simulink model "OEW_PMSM_180_SVPWM_FOC"  (R2022b)
settings: Solver=FixedStepAuto  StartTime=0.0  StopTime=0.3  FixedStep=Ts  RelTol=1e-3
model workspace (MAT data in the model file):
  B = Simulink.Parameter
  B.Value = 0.002
  B.DataType = 'auto'
  B.Complexity = 'real'
  B.Dimensions = [1 1]
  J = Simulink.Parameter
  J.Value = 0.001
  J.DataType = 'auto'
  J.Complexity = 'real'
  J.Dimensions = [1 1]
  L0 = Simulink.Parameter
  L0.Value = 0.001
  L0.DataType = 'auto'
  L0.Complexity = 'real'
  L0.Dimensions = [1 1]
  Ld = Simulink.Parameter
  Ld.Value = 0.00176
  Ld.DataType = 'auto'
  Ld.Complexity = 'real'
  Ld.Dimensions = [1 1]
  Lq = Simulink.Parameter
  Lq.Value = 0.00176
  Lq.DataType = 'auto'
  Lq.Complexity = 'real'
  Lq.Dimensions = [1 1]
  Rs = Simulink.Parameter
  Rs.Value = 0.2
  Rs.DataType = 'auto'
  Rs.Complexity = 'real'
  Rs.Dimensions = [1 1]
  flux = Simulink.Parameter
  flux.Value = 0.1688
  flux.DataType = 'auto'
  flux.Complexity = 'real'
  flux.Dimensions = [1 1]
  flux_3 = Simulink.Parameter
  flux_3.Value = 0.006
  flux_3.DataType = 'auto'
  flux_3.Complexity = 'real'
  flux_3.Dimensions = [1 1]
  pn = Simulink.Parameter
  pn.Value = 4
  pn.DataType = 'auto'
  pn.Complexity = 'real'
  pn.Dimensions = [1 1]
undefined symbols (not defined in the file): DiscIntNeverNeededParam, Tpwm, Ts, Tsample, Tspeed, Udc
libraries: spsControlledCurrentSourceLib x3, spsVoltageMeasurementLib x3, slpidlib x3, spsUniversalBridgeLib x2, simulink x1, spsDCVoltageSourceLib x1, spsSecondOrderFilterLib x1, sps_lib x1
settings Model: DataDictionary=OEW_PMSM_180_SVPWM_FOC.sldd  Creator=SSC  LastModifiedBy=SSC

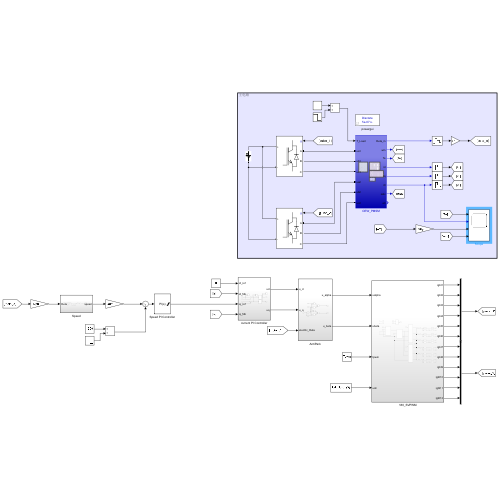
[thumbnail: Simulink's stored preview of the top-level diagram]
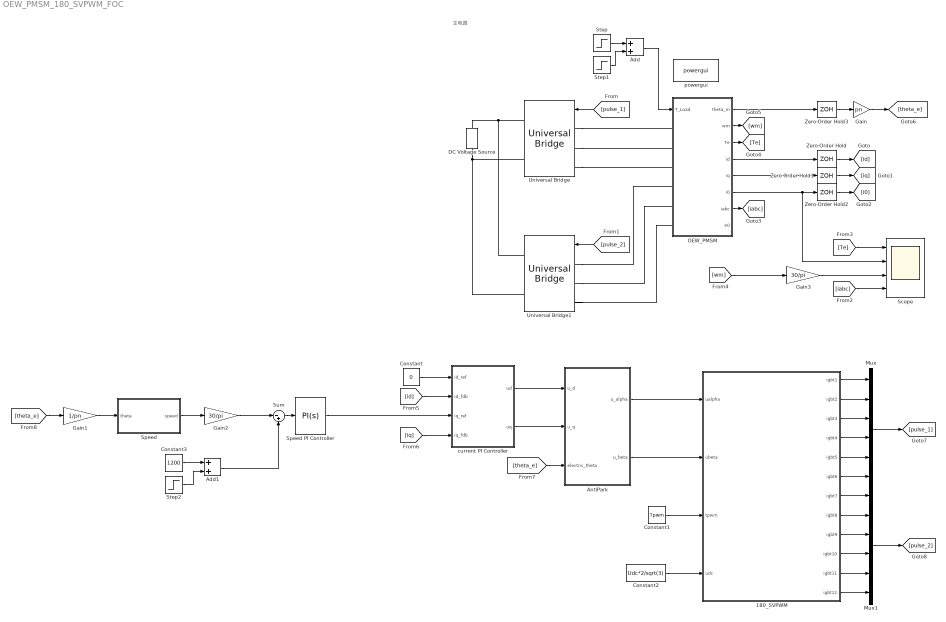
== system OEW_PMSM_180_SVPWM_FOC ==
  note: 主电路
  180_SVPWM : Subsystem
  Add : Sum
  Add1 : Sum
  AntiPark : Subsystem
  Constant : Constant  Value=0
  Constant1 : Constant  Value=Tpwm
  Constant2 : Constant  Value=Udc*2/sqrt(3)
  Constant3 : Constant  Value=1200
  DC Voltage Source : spsDCVoltageSourceLib/DC Voltage Source  Amplitude=Udc  Measurements=None
  Gain : Gain  Gain=pn
  Gain1 : Gain  Gain=1/pn
  Gain2 : Gain  Gain=30/pi
  Gain3 : Gain  Gain=30/pi
  Mux : Mux  Inputs=6
  Mux1 : Mux  Inputs=6
  OEW_PMSM : Subsystem
  Scope : Scope  NumInputPorts=4
  Speed : Subsystem
  Speed PI Controller : slpidlib/PID Controller  Controller=PI  Form=Parallel  TimeDomain=Continuous-time  UseExternalTs=off  SampleTime=1e-4  IntegratorMethod=Forward Euler  FilterMethod=Forward Euler  ControllerParametersSource=internal  P=0.1  I=40  UseKiTs=off  D=0  N=100  UseFilter=on  TunerSelectOption=Transfer Function Based (PID Tuner App)  InitialConditionSource=internal  InitialConditionForIntegrator=0  InitialConditionForFilter=0  DifferentiatorICPrevScaledInput=0  ExternalReset=none  TrackingMode=off  Kt=1  LimitOutput=on  SatLimitsSource=internal  UpperSaturationLimit=14  LowerSaturationLimit=-14  LinearizeAsGain=on  AntiWindupMode=clamping  Kb=1  LimitIntegrator=off  UpperIntegratorSaturationLimit=inf  LowerIntegratorSaturationLimit=-inf  POutMin=[]  POutMax=[]  IOutMin=[]  IOutMax=[]  DOutMin=[]  DOutMax=[]  NOutMin=[]  NOutMax=[]  SumOutMin=[]  SumOutMax=[]  SaturationOutMin=[]  SaturationOutMax=[]  PParamMin=[]  PParamMax=[]  IParamMin=[]  IParamMax=[]  DParamMin=[]  DParamMax=[]  NParamMin=[]  NParamMax=[]  KbParamMin=[]  KbParamMax=[]  KtParamMin=[]  KtParamMax=[]  KbOutMin=[]  KbOutMax=[]  KtOutMin=[]  KtOutMax=[]  IntegratorOutMin=[]  IntegratorOutMax=[]  FilterOutMin=[]  FilterOutMax=[]  SumI1OutMin=[]  SumI1OutMax=[]  SumI2OutMin=[]  SumI2OutMax=[]  SumI3OutMin=[]  SumI3OutMax=[]  SumI4OutMin=[]  SumI4OutMax=[]  SumDOutMin=[]  SumDOutMax=[]  DifferentiatorOutMin=[]  DifferentiatorOutMax=[]  FilterDiffOutCoefMin=[]  FilterDiffOutCoefMax=[]  ReciprocalOutMin=[]  ReciprocalOutMax=[]  SumDenOutMin=[]  SumDenOutMax=[]  SumNumOutMin=[]  SumNumOutMax=[]  DivideOutMin=[]  DivideOutMax=[]  UdiffTsProdOutMin=[]  UdiffTsProdOutMax=[]  NTsProdOutMin=[]  NTsProdOutMax=[]  UintegralTsProdOutMin=[]  UintegralTsProdOutMax=[]  UngainTsProdOutMin=[]  UngainTsProdOutMax=[]  ClampingZeroOutDataTypeStr=Inherit: Inherit via back propagation  ClampingZeroOutMin=[]  ClampingZeroOutMax=[]  FilterDenConstantOutDataTypeStr=Inherit: Inherit via back propagation  FilterDenConstantOutMin=[]  FilterDenConstantOutMax=[]  PCopyOutDataTypeStr=Inherit: Inherit via back propagation  PCopyOutMin=[]  PCopyOutMax=[]  NCopyOutDataTypeStr=Inherit: Inherit via back propagation  NCopyOutMin=[]  NCopyOutMax=[]  IntegratorContinuousStateAttributes=''  IntegratorStateMustResolveToSignalObject=off  IntegratorRTWStateStorageClass=Auto  FilterContinuousStateAttributes=''  FilterStateMustResolveToSignalObject=off  FilterRTWStateStorageClass=Auto  ParallelPVariant=InternalParameters  IdealPVariant=Disabled  IVariant=InternalParameters  DVariant=Disabled  IntegratorVariant=Continuous  SatVariant=Enabled  AWVariant=ContClampingParallel  PCopyVariant=Disabled  TRVariant=Disabled  FdbkBlocksVariant=Forward  IdealPFdbkVariant=Disabled  SatFdbkVariant=Disabled  DerivativeFilterVariant=Disabled  NVariant=Disabled  NCopyVariant=Disabled_SignalSpec  FilterICVariant=Disabled  IntegratorICVariant=InternalICs  ExternalResetVariant=Disabled  TRSumVariant=Passthrough  SumFdbkVariant=Disabled  SumVariant=Sum_PI  TsampFilterVariant=InternalTs  TsampNgainVariant=Passthrough  TsampIntegralVariant=Passthrough  ExternalSaturationOutDataTypeStr=Inherit: Same as second input
  Step : Step  Time=0.05  After=12  SampleTime=0
  Step1 : Step  Time=0.12  After=-6  SampleTime=0
  Step2 : Step  Time=0.15  After=-600  SampleTime=0
  Sum : Sum  Inputs=|-+
  Universal Bridge : spsUniversalBridgeLib/Universal Bridge  Arms=3  SnubberResistance=1e5  SnubberCapacitance=inf  Device=IGBT / Diodes  Ron=1e-3  Lon=0  ForwardVoltages="[  0  0  ]"  ForwardVoltage=0  GTOparameters=[ 10e-6 , 20e-6 ]  IGBTparameters=[ 1e-6 , 2e-6 ]  Measurements=None  Measurements_2=None  converterType=Rectifier
  Universal Bridge1 : spsUniversalBridgeLib/Universal Bridge  Arms=3  SnubberResistance=1e5  SnubberCapacitance=inf  Device=IGBT / Diodes  Ron=1e-3  Lon=0  ForwardVoltages="[  0  0  ]"  ForwardVoltage=0  GTOparameters=[ 10e-6 , 20e-6 ]  IGBTparameters=[ 1e-6 , 2e-6 ]  Measurements=None  Measurements_2=None  converterType=Rectifier
  Zero-Order Hold{,1..3} (4 alike) : ZeroOrderHold  SampleTime=Tsample
  current PI Controller : Subsystem
  powergui : sps_lib/powergui  Priority=1  SimulationMode=Discrete  SampleTime=Ts  frequency=60  Iterations=50  frequencyindice=0  Pbase=100e6  ErrMax=1e-4  UnitsV=kV  UnitsW=MW  buscounter=0  FunctionMessages=off  echomessages=off  EnableUseOfTLC=off  CurrentSourceSwitches=off  DisableSnubberDevices=off  DisableRonSwitches=off  DisableVfSwitches=off  DisplayEquations=off  AutomaticDiscreteSolvers=off  SolverType=Tustin/Backward Euler (TBE)  Interpol=off  ExternalGateDelay=off  methode=off  Ts=100  x0status=blocks  SPID=on  SwTol=0  HookPort=off  NonlinearTolerance=1e-4  nMaxIteration=100  ContinueOnMaxIteration=off  RestoreLinks=warning  ResistiveCurrentMeasurement=off  Frange=[0:2:500]  Ylog=off  Xlog=on  ShowGrid=off  save=off  variable=ZData  structure=0  ZoomFFT=off  StartTime=0.0  cycles=1  DisplayStyle=1  fundamental=60  FreqAxis=off  MaxFrequency=1000  frequencyindicesteady=1  RmsSteady=1  display=off
  wires:
  [pulse_1] -> Universal Bridge/1
  [pulse_2] -> Universal Bridge1/1
  OEW_PMSM/4(id) -> Zero-Order Hold/1
  OEW_PMSM/5(iq) -> Zero-Order Hold1/1
  OEW_PMSM/6(i0) -> Scope/2, Zero-Order Hold2/1
  Zero-Order Hold/1 -> [id]
  Zero-Order Hold1/1 -> [iq]
  Zero-Order Hold2/1 -> [i0]
  OEW_PMSM/7(iabc) -> [iabc]
  [iabc] -> Scope/4
  OEW_PMSM/3(Te) -> [Te]
  [Te] -> Scope/1
  OEW_PMSM/2(wm) -> [wm]
  [wm] -> Gain3/1
  OEW_PMSM/1(theta_m) -> Zero-Order Hold3/1
  Zero-Order Hold3/1 -> Gain/1
  Gain/1 -> [theta_e]
  Step1/1 -> Add/2
  Step/1 -> Add/1
  Add/1 -> OEW_PMSM/1(T_Load)
  Constant/1 -> current PI Controller/1(id_ref)
  [id] -> current PI Controller/2(id_fdb)
  [iq] -> current PI Controller/4(iq_fdb)
  current PI Controller/1(ud) -> AntiPark/1(u_d)
  current PI Controller/2(uq) -> AntiPark/2(u_q)
  [theta_e] -> AntiPark/3(electric_theta)
  AntiPark/1(u_alpha) -> 180_SVPWM/1(ualpha)
  AntiPark/2(u_beta) -> 180_SVPWM/2(ubeta)
  180_SVPWM/5(igbt5) -> Mux/5
  180_SVPWM/6(igbt6) -> Mux/6
  180_SVPWM/4(igbt4) -> Mux/4
  180_SVPWM/3(igbt3) -> Mux/3
  180_SVPWM/2(igbt2) -> Mux/2
  180_SVPWM/1(igbt1) -> Mux/1
  Constant1/1 -> 180_SVPWM/3(tpwm)
  Constant2/1 -> 180_SVPWM/4(udc)
  Mux/1 -> [pulse_1]
  180_SVPWM/7(igbt7) -> Mux1/1
  Mux1/1 -> [pulse_2]
  180_SVPWM/11(igbt11) -> Mux1/5
  180_SVPWM/8(igbt8) -> Mux1/2
  180_SVPWM/10(igbt10) -> Mux1/4
  180_SVPWM/9(igbt9) -> Mux1/3
  180_SVPWM/12(igbt12) -> Mux1/6
  Gain1/1 -> Speed/1(theta)
  [theta_e] -> Gain1/1
  Speed/1(speed) -> Gain2/1
  Gain2/1 -> Sum/1
  Constant3/1 -> Add1/1
  Sum/1 -> Speed PI Controller/1
  Add1/1 -> Sum/2
  Step2/1 -> Add1/2
  Speed PI Controller/1 -> current PI Controller/3(iq_ref)
  Gain3/1 -> Scope/3
  connections:
  Universal Bridge/LConn1 -- OEW_PMSM/LConn1
  Universal Bridge/LConn2 -- OEW_PMSM/LConn2
  Universal Bridge/LConn3 -- OEW_PMSM/LConn3
  Universal Bridge1/LConn1 -- OEW_PMSM/LConn4
  Universal Bridge1/LConn2 -- OEW_PMSM/LConn5
  Universal Bridge1/LConn3 -- OEW_PMSM/LConn6
  DC Voltage Source/LConn1 -- Universal Bridge/RConn2 -- Universal Bridge1/RConn2
  Universal Bridge1/RConn1 -- Universal Bridge/RConn1 -- DC Voltage Source/RConn1

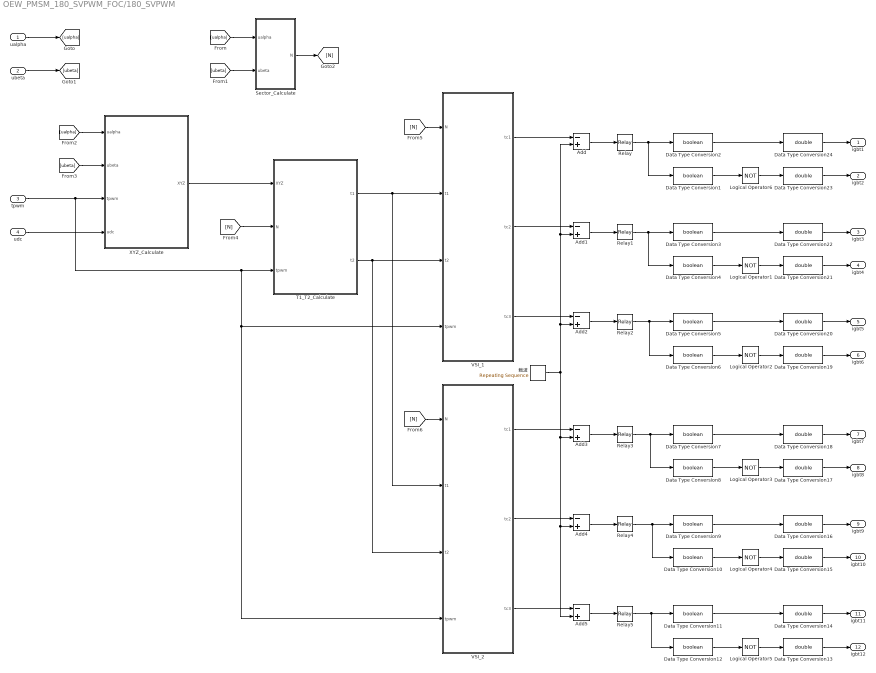
== system OEW_PMSM_180_SVPWM_FOC/180_SVPWM ==
  ualpha : Inport
  ubeta : Inport  Port=2
  tpwm : Inport  Port=3
  udc : Inport  Port=4
  Add{,1..5} (6 alike) : Sum  Inputs=-+
  Data Type Conversion{1..12} (12 alike) : DataTypeConversion  OutDataTypeStr=boolean  SaturateOnIntegerOverflow=off  RndMeth=Floor
  Data Type Conversion{13..24} (12 alike) : DataTypeConversion  OutDataTypeStr=double  SaturateOnIntegerOverflow=off  RndMeth=Floor
  Logical Operator{1..6} (6 alike) : Logic  Operator=NOT  AllPortsSameDT=off  OutDataTypeStr=boolean
  Relay{,1..5} (6 alike) : Relay
  Sector_Calculate : Subsystem
  T1_T2_Calculate : Subsystem
  VSI_1 : Subsystem
  VSI_2 : Subsystem
  XYZ_Calculate : Subsystem
  载波 : simulink/Sources/Repeating Sequence  rep_seq_t=[0 0.5*(1e-4) 1e-4]  rep_seq_y=[0 0.5*(1e-4) 0]
  igbt1 : Outport
  igbt2 : Outport  Port=2
  igbt3 : Outport  Port=3
  igbt4 : Outport  Port=4
  igbt5 : Outport  Port=5
  igbt6 : Outport  Port=6
  igbt7 : Outport  Port=7
  igbt8 : Outport  Port=8
  igbt9 : Outport  Port=9
  igbt10 : Outport  Port=10
  igbt11 : Outport  Port=11
  igbt12 : Outport  Port=12
  wires:
  [ubeta] -> XYZ_Calculate/2(ubeta)
  Relay5/1 -> Data Type Conversion11/1, Data Type Conversion12/1
  Relay2/1 -> Data Type Conversion5/1, Data Type Conversion6/1
  Add2/1 -> Relay2/1
  VSI_1/1(tc1) -> Add/1
  T1_T2_Calculate/2(t2) -> VSI_1/3(t2), VSI_2/3(t2)
  VSI_2/1(tc1) -> Add3/1
  [N] -> VSI_1/1(N)
  Relay1/1 -> Data Type Conversion3/1, Data Type Conversion4/1
  Add3/1 -> Relay3/1
  Add4/1 -> Relay4/1
  Sector_Calculate/1(N) -> [N]
  [ubeta] -> Sector_Calculate/2(ubeta)
  udc/1 -> XYZ_Calculate/4(udc)
  Relay4/1 -> Data Type Conversion9/1, Data Type Conversion10/1
  [N] -> T1_T2_Calculate/2(N)
  载波/1 -> Add/2, Add1/2, Add2/2, Add5/2, Add4/2, Add3/2
  Add/1 -> Relay/1
  [ualpha] -> Sector_Calculate/1(ualpha)
  T1_T2_Calculate/1(t1) -> VSI_1/2(t1), VSI_2/2(t1)
  tpwm/1 -> VSI_2/4(tpwm), VSI_1/4(tpwm), T1_T2_Calculate/3(tpwm), XYZ_Calculate/3(tpwm)
  Logical Operator1/1 -> Data Type Conversion21/1
  Relay/1 -> Data Type Conversion2/1, Data Type Conversion1/1
  XYZ_Calculate/1(XYZ) -> T1_T2_Calculate/1(XYZ)
  Logical Operator2/1 -> Data Type Conversion19/1
  [N] -> VSI_2/1(N)
  Relay3/1 -> Data Type Conversion7/1, Data Type Conversion8/1
  Logical Operator6/1 -> Data Type Conversion23/1
  [ualpha] -> XYZ_Calculate/1(ualpha)
  Logical Operator5/1 -> Data Type Conversion13/1
  Logical Operator4/1 -> Data Type Conversion15/1
  VSI_1/2(tc2) -> Add1/1
  Add5/1 -> Relay5/1
  VSI_2/3(tc3) -> Add5/1
  Add1/1 -> Relay1/1
  VSI_2/2(tc2) -> Add4/1
  VSI_1/3(tc3) -> Add2/1
  Logical Operator3/1 -> Data Type Conversion17/1
  Data Type Conversion2/1 -> Data Type Conversion24/1
  Data Type Conversion1/1 -> Logical Operator6/1
  Data Type Conversion3/1 -> Data Type Conversion22/1
  Data Type Conversion4/1 -> Logical Operator1/1
  Data Type Conversion5/1 -> Data Type Conversion20/1
  Data Type Conversion6/1 -> Logical Operator2/1
  Data Type Conversion7/1 -> Data Type Conversion18/1
  Data Type Conversion8/1 -> Logical Operator3/1
  Data Type Conversion9/1 -> Data Type Conversion16/1
  Data Type Conversion10/1 -> Logical Operator4/1
  Data Type Conversion11/1 -> Data Type Conversion14/1
  Data Type Conversion12/1 -> Logical Operator5/1
  Data Type Conversion13/1 -> igbt12/1
  Data Type Conversion14/1 -> igbt11/1
  Data Type Conversion15/1 -> igbt10/1
  Data Type Conversion16/1 -> igbt9/1
  Data Type Conversion17/1 -> igbt8/1
  Data Type Conversion18/1 -> igbt7/1
  Data Type Conversion19/1 -> igbt6/1
  Data Type Conversion20/1 -> igbt5/1
  Data Type Conversion21/1 -> igbt4/1
  Data Type Conversion22/1 -> igbt3/1
  Data Type Conversion23/1 -> igbt2/1
  Data Type Conversion24/1 -> igbt1/1
  ualpha/1 -> [ualpha]
  ubeta/1 -> [ubeta]

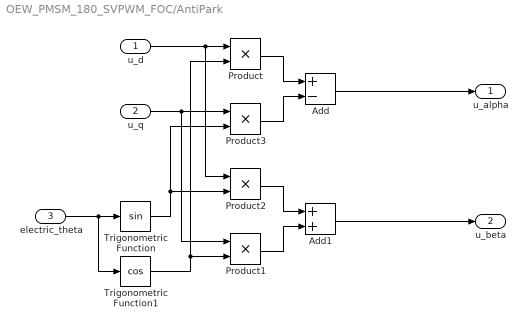
== system OEW_PMSM_180_SVPWM_FOC/AntiPark ==
  u_d : Inport
  u_q : Inport  Port=2
  electric_theta : Inport  Port=3
  Add : Sum  Inputs=+-
  Add1 : Sum
  Product{,1..3} (4 alike) : Product
  Trigonometric Function : Trigonometry
  Trigonometric Function1 : Trigonometry  Operator=cos
  u_alpha : Outport
  u_beta : Outport  Port=2
  wires:
  electric_theta/1 -> Trigonometric Function1/1, Trigonometric Function/1
  u_d/1 -> Product2/1, Product/1
  Trigonometric Function1/1 -> Product/2, Product1/2
  u_q/1 -> Product1/1, Product3/1
  Trigonometric Function/1 -> Product2/2, Product3/2
  Product/1 -> Add/1
  Product3/1 -> Add/2
  Add/1 -> u_alpha/1
  Product2/1 -> Add1/1
  Product1/1 -> Add1/2
  Add1/1 -> u_beta/1

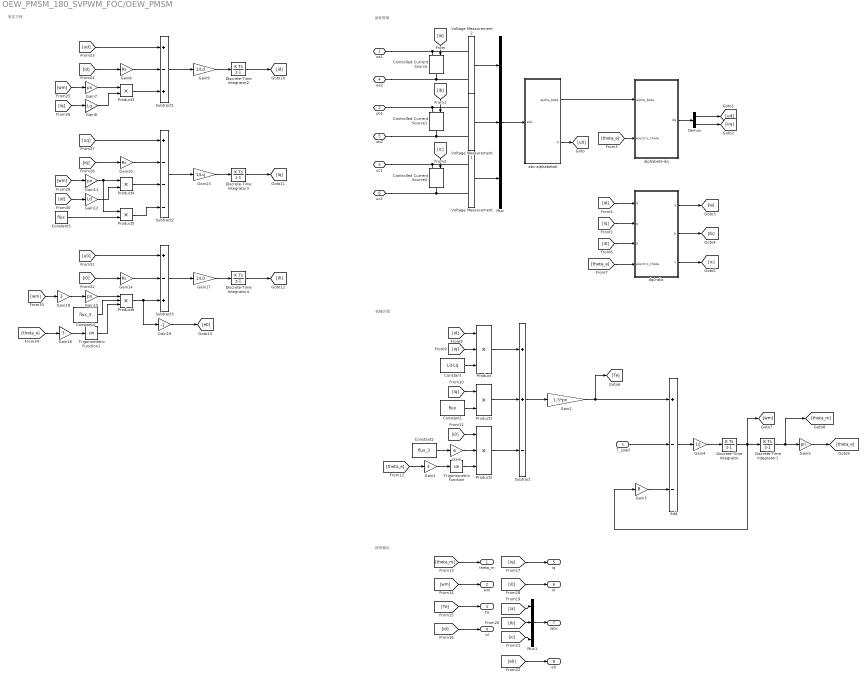
== system OEW_PMSM_180_SVPWM_FOC/OEW_PMSM ==
  note: 电压方程
  note: 信号输出
  note: 机械方程
  note: 坐标变换
  T_Load : Inport
  Add : Sum  Inputs=+--
  Constant : Constant  Value=Ld-Lq
  Constant1 : Constant  Value=flux
  Constant2 : Constant  Value=flux_3
  Constant3 : Constant  Value=flux
  Constant4 : Constant  Value=flux_3
  Controlled Current Source : spsControlledCurrentSourceLib/Controlled Current Source  Initialize=on  Source_Type=AC  Amplitude=0  Phase=0  Frequency=0  Measurements=None
  Controlled Current Source1 : spsControlledCurrentSourceLib/Controlled Current Source  Initialize=on  Source_Type=AC  Amplitude=0  Phase=0  Frequency=0  Measurements=None
  Controlled Current Source2 : spsControlledCurrentSourceLib/Controlled Current Source  Initialize=on  Source_Type=AC  Amplitude=0  Phase=0  Frequency=0  Measurements=None
  Demux : Demux  Outputs=2
  Discrete-Time Integrator{,1..4} (5 alike) : DiscreteIntegrator  SampleTime=Ts  ICPrevOutput=DiscIntNeverNeededParam  ICPrevScaledInput=DiscIntNeverNeededParam
  Gain : Gain  Gain=6
  Gain1 : Gain  Gain=3
  Gain10 : Gain  Gain=Rs
  Gain{5,7,11,15} (4 alike) : Gain  Gain=pn
  Gain12 : Gain  Gain=Ld
  Gain13 : Gain  Gain=1/Lq
  Gain14 : Gain  Gain=Rs
  Gain16 : Gain  Gain=3
  Gain17 : Gain  Gain=1/L0
  Gain18 : Gain  Gain=3
  Gain19 : Gain  Gain=-1
  Gain2 : Gain  Gain=1.5*pn
  Gain3 : Gain  Gain=B
  Gain4 : Gain  Gain=1/J
  Gain6 : Gain  Gain=Rs
  Gain8 : Gain  Gain=Lq
  Gain9 : Gain  Gain=1/Ld
  Mux : Mux  Inputs=3
  Mux1 : Mux  Inputs=3
  Product : Product  Inputs=3
  Product{1,3..5} (4 alike) : Product
  Product2 : Product  Inputs=3
  Product6 : Product  Inputs=3
  Subtract : Sum  Inputs=++-
  Subtract1 : Sum  Inputs=+-+
  Subtract2 : Sum  Inputs=+---
  Subtract3 : Sum  Inputs=+-+
  Trigonometric Function : Trigonometry
  Trigonometric Function1 : Trigonometry
  Voltage Measurement : spsVoltageMeasurementLib/Voltage Measurement  PhasorSimulation=off  OutputType=Complex  PSBequivalent=0
  Voltage Measurement1 : spsVoltageMeasurementLib/Voltage Measurement  PhasorSimulation=off  OutputType=Complex  PSBequivalent=0
  Voltage Measurement2 : spsVoltageMeasurementLib/Voltage Measurement  PhasorSimulation=off  OutputType=Complex  PSBequivalent=0
  abc-alphabeta0 : Subsystem
  alphabeta-dq : Subsystem
  dq0-abc : Subsystem
  ua1 : PMIOPort  Side=Left
  ub1 : PMIOPort  Port=2  Side=Left
  uc1 : PMIOPort  Port=3  Side=Left
  ua2 : PMIOPort  Port=4  Side=Left
  ub2 : PMIOPort  Port=5  Side=Left
  uc2 : PMIOPort  Port=6  Side=Left
  theta_m : Outport
  wm : Outport  Port=2
  Te : Outport  Port=3
  id : Outport  Port=4
  iq : Outport  Port=5
  i0 : Outport  Port=6
  iabc : Outport  Port=7
  e0 : Outport  Port=8
  wires:
  [id] -> Gain12/1
  [id] -> Product/1
  [iq] -> Product/2
  [i0] -> Gain14/1
  alphabeta-dq/1(dq) -> Demux/1
  Gain12/1 -> Product4/2
  Gain19/1 -> [e0]
  [ia] -> Mux1/1
  [iq] -> Gain8/1
  abc-alphabeta0/1(alpha_beta) -> alphabeta-dq/1(alpha_beta)
  Product3/1 -> Subtract1/3
  Subtract2/1 -> Gain13/1
  Gain6/1 -> Subtract1/2
  Product1/1 -> Subtract/2
  Demux/1 -> [ud]
  [theta_e] -> alphabeta-dq/2(electric_theta)
  Gain13/1 -> Discrete-Time Integrator3/1
  Constant1/1 -> Product1/2
  Subtract1/1 -> Gain9/1
  Voltage Measurement1/1 -> Mux/2
  Gain11/1 -> Product5/1, Product4/1
  [ic] -> Controlled Current Source2/1
  dq0-abc/1(a) -> [ia]
  Mux/1 -> abc-alphabeta0/1(abc)
  [iq] -> Gain10/1
  Gain4/1 -> Discrete-Time Integrator/1
  [ib] -> Controlled Current Source1/1
  Demux/2 -> [uq]
  [theta_e] -> Gain16/1
  [ic] -> Mux1/3
  Voltage Measurement/1 -> Mux/3
  Gain3/1 -> Add/3
  Product4/1 -> Subtract2/3
  [iq] -> iq/1
  Gain16/1 -> Trigonometric Function1/1
  [ia] -> Controlled Current Source/1
  Gain1/1 -> Trigonometric Function/1
  abc-alphabeta0/2(0) -> [u0]
  dq0-abc/3(c) -> [ic]
  dq0-abc/2(b) -> [ib]
  T_Load/1 -> Add/2
  [ud] -> Subtract1/1
  Discrete-Time Integrator3/1 -> [iq]
  Voltage Measurement2/1 -> Mux/1
  Constant3/1 -> Product5/2
  Subtract3/1 -> Gain17/1
  Constant/1 -> Product/3
  [iq] -> dq0-abc/2(q)
  [uq] -> Subtract2/1
  Add/1 -> Gain4/1
  [theta_e] -> dq0-abc/4(electric_theta)
  [i0] -> dq0-abc/3(0)
  Product6/1 -> Subtract3/3, Gain19/1
  [id] -> dq0-abc/1(d)
  [wm] -> wm/1
  Discrete-Time Integrator/1 -> Discrete-Time Integrator1/1, Gain3/1, [wm]
  [iq] -> Product1/1
  [wm] -> Gain7/1
  Product/1 -> Subtract/1
  Gain10/1 -> Subtract2/2
  [wm] -> Gain11/1
  Product5/1 -> Subtract2/4
  Constant4/1 -> Product6/2
  Mux1/1 -> iabc/1
  Gain18/1 -> Gain15/1
  Gain5/1 -> [theta_e]
  Trigonometric Function1/1 -> Product6/3
  Gain9/1 -> Discrete-Time Integrator2/1
  Gain7/1 -> Product3/1
  Trigonometric Function/1 -> Product2/3
  Discrete-Time Integrator1/1 -> Gain5/1, [theta_m]
  [ib] -> Mux1/2
  [theta_e] -> Gain1/1
  Gain8/1 -> Product3/2
  [Te] -> Te/1
  Product2/1 -> Subtract/3
  [i0] -> Product2/1
  Discrete-Time Integrator2/1 -> [id]
  [id] -> Gain6/1
  Gain/1 -> Product2/2
  Gain2/1 -> Add/1, [Te]
  Constant2/1 -> Gain/1
  Subtract/1 -> Gain2/1
  [theta_m] -> theta_m/1
  Discrete-Time Integrator4/1 -> [i0]
  Gain17/1 -> Discrete-Time Integrator4/1
  Gain15/1 -> Product6/1
  [u0] -> Subtract3/1
  Gain14/1 -> Subtract3/2
  [wm] -> Gain18/1
  [i0] -> i0/1
  [id] -> id/1
  [e0] -> e0/1
  connections:
  Voltage Measurement2/LConn2 -- ua2/RConn1 -- Controlled Current Source/RConn1
  Voltage Measurement1/LConn2 -- ub2/RConn1 -- Controlled Current Source1/RConn1
  Voltage Measurement2/LConn1 -- ua1/RConn1 -- Controlled Current Source/LConn1
  Voltage Measurement/LConn2 -- uc2/RConn1 -- Controlled Current Source2/RConn1
  Voltage Measurement1/LConn1 -- ub1/RConn1 -- Controlled Current Source1/LConn1
  Voltage Measurement/LConn1 -- uc1/RConn1 -- Controlled Current Source2/LConn1

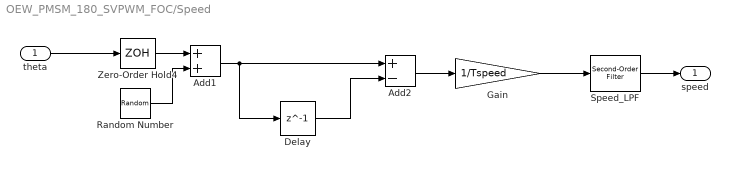
== system OEW_PMSM_180_SVPWM_FOC/Speed ==
  theta : Inport
  Add1 : Sum
  Add2 : Sum  Inputs=+-
  Delay : Delay  DelayLength=1  InitialCondition=0  SampleTime=Tspeed
  Gain : Gain  Gain=1/Tspeed
  Random Number : RandomNumber  Mean=2.5e-10  Variance=2.5e-10  SampleTime=Tspeed
  Speed_LPF : spsSecondOrderFilterLib/Second-Order Filter  FilterType=Lowpass  Fo=500  Zeta=0.707  Ts=Tspeed  Initialize=off  Vac_Init="[0,  0,  60]"  Vdc_Init=0  PlotResponse=off  FreqRange=[0, 500, 1]
      settings: LibrarySourceBlock=|
      | sps_lib/Control/Filters/Second-Order
      | Filter
  Zero-Order Hold4 : ZeroOrderHold  SampleTime=Tspeed
  speed : Outport
  wires:
  Zero-Order Hold4/1 -> Add1/1
  Random Number/1 -> Add1/2
  theta/1 -> Zero-Order Hold4/1
  Speed_LPF/1 -> speed/1
  Add2/1 -> Gain/1
  Gain/1 -> Speed_LPF/1
  Add1/1 -> Delay/1, Add2/1
  Delay/1 -> Add2/2

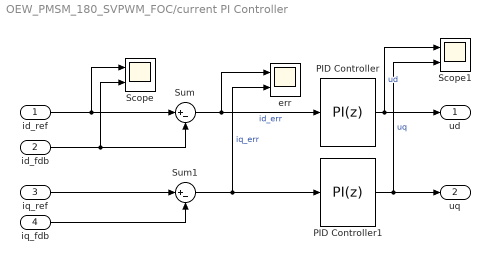
== system OEW_PMSM_180_SVPWM_FOC/current PI Controller ==
  id_ref : Inport
  id_fdb : Inport  Port=2
  iq_ref : Inport  Port=3
  iq_fdb : Inport  Port=4
  PID Controller : slpidlib/PID Controller  Controller=PI  Form=Parallel  TimeDomain=Discrete-time  UseExternalTs=off  SampleTime=Tsample  IntegratorMethod=Forward Euler  FilterMethod=Forward Euler  ControllerParametersSource=internal  P=5.5292  I=628.32  UseKiTs=off  D=0  N=100  UseFilter=on  TunerSelectOption=Transfer Function Based (PID Tuner App)  InitialConditionSource=internal  InitialConditionForIntegrator=0  InitialConditionForFilter=0  DifferentiatorICPrevScaledInput=0  ExternalReset=none  TrackingMode=off  Kt=1  LimitOutput=on  SatLimitsSource=internal  UpperSaturationLimit=Udc  LowerSaturationLimit=-Udc  LinearizeAsGain=on  AntiWindupMode=clamping  Kb=1  LimitIntegrator=off  UpperIntegratorSaturationLimit=inf  LowerIntegratorSaturationLimit=-inf  POutMin=[]  POutMax=[]  IOutMin=[]  IOutMax=[]  DOutMin=[]  DOutMax=[]  NOutMin=[]  NOutMax=[]  SumOutMin=[]  SumOutMax=[]  SaturationOutMin=[]  SaturationOutMax=[]  PParamMin=[]  PParamMax=[]  IParamMin=[]  IParamMax=[]  DParamMin=[]  DParamMax=[]  NParamMin=[]  NParamMax=[]  KbParamMin=[]  KbParamMax=[]  KtParamMin=[]  KtParamMax=[]  KbOutMin=[]  KbOutMax=[]  KtOutMin=[]  KtOutMax=[]  IntegratorOutMin=[]  IntegratorOutMax=[]  FilterOutMin=[]  FilterOutMax=[]  SumI1OutMin=[]  SumI1OutMax=[]  SumI2OutMin=[]  SumI2OutMax=[]  SumI3OutMin=[]  SumI3OutMax=[]  SumI4OutMin=[]  SumI4OutMax=[]  SumDOutMin=[]  SumDOutMax=[]  DifferentiatorOutMin=[]  DifferentiatorOutMax=[]  FilterDiffOutCoefMin=[]  FilterDiffOutCoefMax=[]  ReciprocalOutMin=[]  ReciprocalOutMax=[]  SumDenOutMin=[]  SumDenOutMax=[]  SumNumOutMin=[]  SumNumOutMax=[]  DivideOutMin=[]  DivideOutMax=[]  UdiffTsProdOutMin=[]  UdiffTsProdOutMax=[]  NTsProdOutMin=[]  NTsProdOutMax=[]  UintegralTsProdOutMin=[]  UintegralTsProdOutMax=[]  UngainTsProdOutMin=[]  UngainTsProdOutMax=[]  ClampingZeroOutDataTypeStr=Inherit: Inherit via back propagation  ClampingZeroOutMin=[]  ClampingZeroOutMax=[]  FilterDenConstantOutDataTypeStr=Inherit: Inherit via back propagation  FilterDenConstantOutMin=[]  FilterDenConstantOutMax=[]  PCopyOutDataTypeStr=Inherit: Inherit via back propagation  PCopyOutMin=[]  PCopyOutMax=[]  NCopyOutDataTypeStr=Inherit: Inherit via back propagation  NCopyOutMin=[]  NCopyOutMax=[]  IntegratorContinuousStateAttributes=''  IntegratorStateMustResolveToSignalObject=off  IntegratorRTWStateStorageClass=Auto  FilterContinuousStateAttributes=''  FilterStateMustResolveToSignalObject=off  FilterRTWStateStorageClass=Auto  ParallelPVariant=InternalParameters  IdealPVariant=Disabled  IVariant=InternalParameters  DVariant=Disabled  IntegratorVariant=Discrete  SatVariant=Enabled  AWVariant=DiscClampingParallel  PCopyVariant=Disabled  TRVariant=Disabled  FdbkBlocksVariant=Forward  IdealPFdbkVariant=Disabled  SatFdbkVariant=Disabled  DerivativeFilterVariant=Disabled  NVariant=Disabled  NCopyVariant=Disabled_SignalSpec  FilterICVariant=Disabled  IntegratorICVariant=InternalICs  ExternalResetVariant=Disabled  TRSumVariant=Passthrough  SumFdbkVariant=Disabled  SumVariant=Sum_PI  TsampFilterVariant=InternalTs  TsampNgainVariant=Passthrough  TsampIntegralVariant=Passthrough  ExternalSaturationOutDataTypeStr=Inherit: Same as second input
  PID Controller1 : slpidlib/PID Controller  Controller=PI  Form=Parallel  TimeDomain=Discrete-time  UseExternalTs=off  SampleTime=Tsample  IntegratorMethod=Forward Euler  FilterMethod=Forward Euler  ControllerParametersSource=internal  P=5.5292  I=628.32  UseKiTs=off  D=0  N=100  UseFilter=on  TunerSelectOption=Transfer Function Based (PID Tuner App)  InitialConditionSource=internal  InitialConditionForIntegrator=0  InitialConditionForFilter=0  DifferentiatorICPrevScaledInput=0  ExternalReset=none  TrackingMode=off  Kt=1  LimitOutput=on  SatLimitsSource=internal  UpperSaturationLimit=Udc  LowerSaturationLimit=-Udc  LinearizeAsGain=on  AntiWindupMode=clamping  Kb=1  LimitIntegrator=off  UpperIntegratorSaturationLimit=inf  LowerIntegratorSaturationLimit=-inf  POutMin=[]  POutMax=[]  IOutMin=[]  IOutMax=[]  DOutMin=[]  DOutMax=[]  NOutMin=[]  NOutMax=[]  SumOutMin=[]  SumOutMax=[]  SaturationOutMin=[]  SaturationOutMax=[]  PParamMin=[]  PParamMax=[]  IParamMin=[]  IParamMax=[]  DParamMin=[]  DParamMax=[]  NParamMin=[]  NParamMax=[]  KbParamMin=[]  KbParamMax=[]  KtParamMin=[]  KtParamMax=[]  KbOutMin=[]  KbOutMax=[]  KtOutMin=[]  KtOutMax=[]  IntegratorOutMin=[]  IntegratorOutMax=[]  FilterOutMin=[]  FilterOutMax=[]  SumI1OutMin=[]  SumI1OutMax=[]  SumI2OutMin=[]  SumI2OutMax=[]  SumI3OutMin=[]  SumI3OutMax=[]  SumI4OutMin=[]  SumI4OutMax=[]  SumDOutMin=[]  SumDOutMax=[]  DifferentiatorOutMin=[]  DifferentiatorOutMax=[]  FilterDiffOutCoefMin=[]  FilterDiffOutCoefMax=[]  ReciprocalOutMin=[]  ReciprocalOutMax=[]  SumDenOutMin=[]  SumDenOutMax=[]  SumNumOutMin=[]  SumNumOutMax=[]  DivideOutMin=[]  DivideOutMax=[]  UdiffTsProdOutMin=[]  UdiffTsProdOutMax=[]  NTsProdOutMin=[]  NTsProdOutMax=[]  UintegralTsProdOutMin=[]  UintegralTsProdOutMax=[]  UngainTsProdOutMin=[]  UngainTsProdOutMax=[]  ClampingZeroOutDataTypeStr=Inherit: Inherit via back propagation  ClampingZeroOutMin=[]  ClampingZeroOutMax=[]  FilterDenConstantOutDataTypeStr=Inherit: Inherit via back propagation  FilterDenConstantOutMin=[]  FilterDenConstantOutMax=[]  PCopyOutDataTypeStr=Inherit: Inherit via back propagation  PCopyOutMin=[]  PCopyOutMax=[]  NCopyOutDataTypeStr=Inherit: Inherit via back propagation  NCopyOutMin=[]  NCopyOutMax=[]  IntegratorContinuousStateAttributes=''  IntegratorStateMustResolveToSignalObject=off  IntegratorRTWStateStorageClass=Auto  FilterContinuousStateAttributes=''  FilterStateMustResolveToSignalObject=off  FilterRTWStateStorageClass=Auto  ParallelPVariant=InternalParameters  IdealPVariant=Disabled  IVariant=InternalParameters  DVariant=Disabled  IntegratorVariant=Discrete  SatVariant=Enabled  AWVariant=DiscClampingParallel  PCopyVariant=Disabled  TRVariant=Disabled  FdbkBlocksVariant=Forward  IdealPFdbkVariant=Disabled  SatFdbkVariant=Disabled  DerivativeFilterVariant=Disabled  NVariant=Disabled  NCopyVariant=Disabled_SignalSpec  FilterICVariant=Disabled  IntegratorICVariant=InternalICs  ExternalResetVariant=Disabled  TRSumVariant=Passthrough  SumFdbkVariant=Disabled  SumVariant=Sum_PI  TsampFilterVariant=InternalTs  TsampNgainVariant=Passthrough  TsampIntegralVariant=Passthrough  ExternalSaturationOutDataTypeStr=Inherit: Same as second input
  Scope : Scope  NumInputPorts=2
  Scope1 : Scope  NumInputPorts=2
  Sum : Sum  Inputs=|+-
  Sum1 : Sum  Inputs=|+-
  err : Scope  NumInputPorts=2
  ud : Outport
  uq : Outport  Port=2
  wires:
  iq_fdb/1 -> Sum1/2
  Sum1/1 -> PID Controller1/1, err/2  "iq_err"
  id_fdb/1 -> Scope/2, Sum/2
  Sum/1 -> err/1, PID Controller/1  "id_err"
  id_ref/1 -> Scope/1, Sum/1
  iq_ref/1 -> Sum1/1
  PID Controller1/1 -> Scope1/2, uq/1  "uq"
  PID Controller/1 -> Scope1/1, ud/1  "ud"

== system OEW_PMSM_180_SVPWM_FOC/180_SVPWM/Sector_Calculate ==
  ualpha : Inport
  ubeta : Inport  Port=2
  MATLAB Function : MATLAB Function  TreatAsAtomicUnit=on
  N : Outport
  wires:
  ualpha/1 -> MATLAB Function/1(ualpha)
  ubeta/1 -> MATLAB Function/2(ubeta)
  MATLAB Function/1(N) -> N/1

== system OEW_PMSM_180_SVPWM_FOC/180_SVPWM/T1_T2_Calculate ==
  XYZ : Inport
  N : Inport  Port=2
  tpwm : Inport  Port=3
  Demux : Demux  Outputs=3
  MATLAB Function : MATLAB Function  TreatAsAtomicUnit=on
  t1 : Outport
  t2 : Outport  Port=2
  wires:
  Demux/2 -> MATLAB Function/2(Y)
  Demux/1 -> MATLAB Function/1(X)
  Demux/3 -> MATLAB Function/3(Z)
  XYZ/1 -> Demux/1
  N/1 -> MATLAB Function/4(N)
  tpwm/1 -> MATLAB Function/5(tpwm)
  MATLAB Function/1(t1) -> t1/1
  MATLAB Function/2(t2) -> t2/1

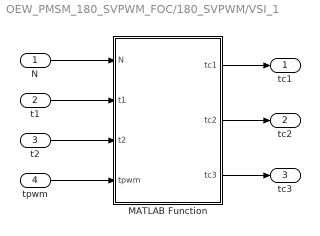
== system OEW_PMSM_180_SVPWM_FOC/180_SVPWM/VSI_1 ==
  N : Inport
  t1 : Inport  Port=2
  t2 : Inport  Port=3
  tpwm : Inport  Port=4
  MATLAB Function : MATLAB Function  TreatAsAtomicUnit=on
  tc1 : Outport
  tc2 : Outport  Port=2
  tc3 : Outport  Port=3
  wires:
  t2/1 -> MATLAB Function/3(t2)
  tpwm/1 -> MATLAB Function/4(tpwm)
  t1/1 -> MATLAB Function/2(t1)
  N/1 -> MATLAB Function/1(N)
  MATLAB Function/1(tc1) -> tc1/1
  MATLAB Function/2(tc2) -> tc2/1
  MATLAB Function/3(tc3) -> tc3/1

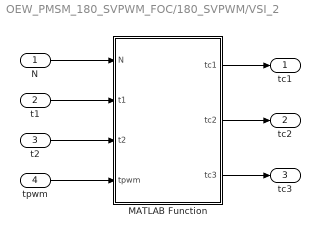
== system OEW_PMSM_180_SVPWM_FOC/180_SVPWM/VSI_2 ==
  N : Inport
  t1 : Inport  Port=2
  t2 : Inport  Port=3
  tpwm : Inport  Port=4
  MATLAB Function : MATLAB Function  TreatAsAtomicUnit=on
  tc1 : Outport
  tc2 : Outport  Port=2
  tc3 : Outport  Port=3
  wires:
  t2/1 -> MATLAB Function/3(t2)
  tpwm/1 -> MATLAB Function/4(tpwm)
  t1/1 -> MATLAB Function/2(t1)
  N/1 -> MATLAB Function/1(N)
  MATLAB Function/1(tc1) -> tc1/1
  MATLAB Function/2(tc2) -> tc2/1
  MATLAB Function/3(tc3) -> tc3/1

== system OEW_PMSM_180_SVPWM_FOC/180_SVPWM/XYZ_Calculate ==
  ualpha : Inport
  ubeta : Inport  Port=2
  tpwm : Inport  Port=3
  udc : Inport  Port=4
  Mux : Mux  Inputs=3
  xyz : MATLAB Function  TreatAsAtomicUnit=on
  XYZ : Outport
  wires:
  ualpha/1 -> xyz/1(ualpha)
  ubeta/1 -> xyz/2(ubeta)
  tpwm/1 -> xyz/3(tpwm)
  udc/1 -> xyz/4(udc)
  Mux/1 -> XYZ/1
  xyz/2(Y) -> Mux/2
  xyz/1(X) -> Mux/1
  xyz/3(Z) -> Mux/3

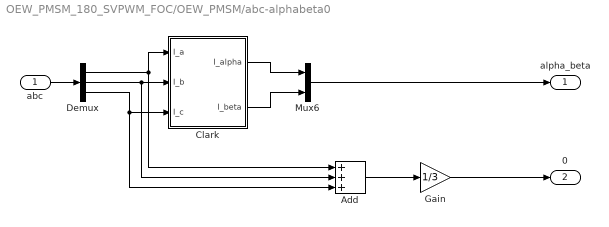
== system OEW_PMSM_180_SVPWM_FOC/OEW_PMSM/abc-alphabeta0 ==
  abc : Inport
  Add : Sum  Inputs=+++
  Clark : Subsystem
  Demux : Demux  Outputs=3
  Gain : Gain  Gain=1/3
  Mux6 : Mux  Inputs=2
  alpha_beta : Outport  VectorParamsAs1DForOutWhenUnconnected=off
  0 : Outport  Port=2  VectorParamsAs1DForOutWhenUnconnected=off
  wires:
  Clark/2(I_beta) -> Mux6/2
  Mux6/1 -> alpha_beta/1
  Demux/3 -> Clark/3(I_c), Add/3
  Clark/1(I_alpha) -> Mux6/1
  abc/1 -> Demux/1
  Demux/2 -> Add/2, Clark/2(I_b)
  Demux/1 -> Clark/1(I_a), Add/1
  Add/1 -> Gain/1
  Gain/1 -> 0/1

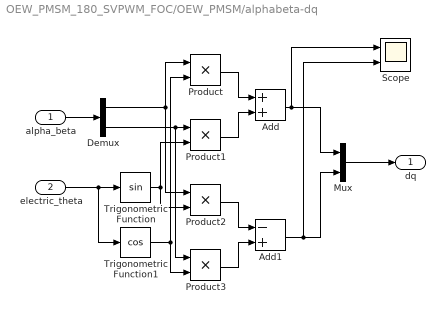
== system OEW_PMSM_180_SVPWM_FOC/OEW_PMSM/alphabeta-dq ==
  alpha_beta : Inport
  electric_theta : Inport  Port=2
  Add : Sum
  Add1 : Sum  Inputs=-+
  Demux : Demux  Outputs=2
  Mux : Mux  Inputs=2
  Product{,1..3} (4 alike) : Product
  Scope : Scope  NumInputPorts=2
  Trigonometric Function : Trigonometry
  Trigonometric Function1 : Trigonometry  Operator=cos
  dq : Outport
  wires:
  electric_theta/1 -> Trigonometric Function1/1, Trigonometric Function/1
  Trigonometric Function1/1 -> Product3/2, Product/2
  Demux/2 -> Product3/1, Product1/1
  Trigonometric Function/1 -> Product2/2, Product1/2
  Product/1 -> Add/1
  Product1/1 -> Add/2
  Product2/1 -> Add1/1
  Product3/1 -> Add1/2
  Add/1 -> Scope/1, Mux/1
  Add1/1 -> Scope/2, Mux/2
  Demux/1 -> Product/1, Product2/1
  alpha_beta/1 -> Demux/1
  Mux/1 -> dq/1

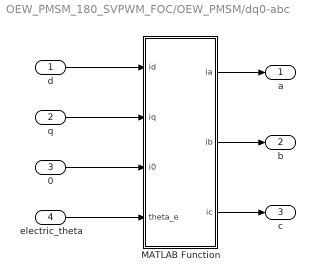
== system OEW_PMSM_180_SVPWM_FOC/OEW_PMSM/dq0-abc ==
  d : Inport
  q : Inport  Port=2
  0 : Inport  Port=3
  electric_theta : Inport  Port=4
  MATLAB Function : MATLAB Function  TreatAsAtomicUnit=on
  a : Outport
  b : Outport  Port=2
  c : Outport  Port=3
  wires:
  d/1 -> MATLAB Function/1(id)
  q/1 -> MATLAB Function/2(iq)
  0/1 -> MATLAB Function/3(i0)
  electric_theta/1 -> MATLAB Function/4(theta_e)
  MATLAB Function/1(ia) -> a/1
  MATLAB Function/2(ib) -> b/1
  MATLAB Function/3(ic) -> c/1

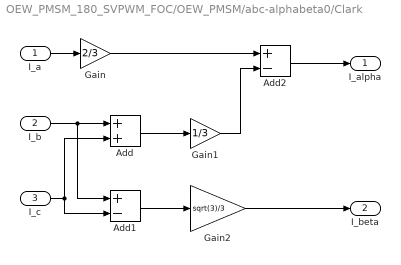
== system OEW_PMSM_180_SVPWM_FOC/OEW_PMSM/abc-alphabeta0/Clark ==
  I_a : Inport
  I_b : Inport  Port=2
  I_c : Inport  Port=3
  Add : Sum
  Add1 : Sum  Inputs=+-
  Add2 : Sum  Inputs=+-
  Gain : Gain  Gain=2/3
  Gain1 : Gain  Gain=1/3
  Gain2 : Gain  Gain=sqrt(3)/3
  I_alpha : Outport
  I_beta : Outport  Port=2
  wires:
  I_a/1 -> Gain/1
  I_b/1 -> Add1/1, Add/1
  I_c/1 -> Add/2, Add1/2
  Add/1 -> Gain1/1
  Add1/1 -> Gain2/1
  Gain/1 -> Add2/1
  Gain1/1 -> Add2/2
  Add2/1 -> I_alpha/1
  Gain2/1 -> I_beta/1

== matlab function OEW_PMSM_180_SVPWM_FOC/180_SVPWM/Sector_Calculate/MATLAB Function ==
  data: ualpha input; N output; ubeta input
function N = fcn(ualpha,ubeta)

u_ref1 = ubeta;
u_ref2 = -0.5 * ubeta + (sqrt(3)/2) * ualpha;
u_ref3 = -0.5 * ubeta - (sqrt(3)/2) * ualpha;

if u_ref1 > 0
    A = 1;
else
    A = 0;
end

if u_ref2 > 0
    B = 1;
else
    B = 0;
end

if u_ref3 > 0
    C = 1;
else
    C = 0;
end

n = A + 2 * B + 4 * C;

if n == 0
    N = 1;
else
    N = n;
end

== matlab function OEW_PMSM_180_SVPWM_FOC/OEW_PMSM/dq0-abc/MATLAB Function ==
  data: id input; ia output; iq input; i0 input; theta_e input; ib output; ic output
function [ia,ib,ic] = fcn(id,iq,i0,theta_e)

ia = id * cos(theta_e) - iq * sin(theta_e) + i0;
ib = id * cos(theta_e - 2*pi/3) - iq * sin(theta_e - 2*pi/3) + i0;
ic = id * cos(theta_e + 2*pi/3) - iq * sin(theta_e + 2*pi/3) + i0;

== matlab function OEW_PMSM_180_SVPWM_FOC/180_SVPWM/XYZ_Calculate/xyz ==
  data: ualpha input; X output; ubeta input; tpwm input; udc input; Y output; Z output
function [X,Y,Z] = fcn(ualpha,ubeta,tpwm,udc)

X = ubeta * tpwm / udc;
Y = (ubeta + (sqrt(3)) * ualpha) * tpwm / (2 * udc);
Z = (ubeta - (sqrt(3)) * ualpha) * tpwm / (2 * udc);

== matlab function OEW_PMSM_180_SVPWM_FOC/180_SVPWM/T1_T2_Calculate/MATLAB Function ==
  data: X input; t1 output; Y input; Z input; N input; tpwm input; t2 output
function [t1, t2] = fcn(X,Y,Z,N,tpwm)

if N == 1
    t_1 = Z;
    t_2 = Y;
elseif N == 2
    t_1 = Y;
    t_2 = -X;
elseif N == 3
    t_1 = -Z;
    t_2 = X;
elseif N == 4
    t_1 = -X;
    t_2 = Z;
elseif N == 5
    t_1 = X;
    t_2 = -Y;
elseif N == 6
    t_1 = -Y;
    t_2 = -Z;
else
    t_1 = Z;
    t_2 = Y;
end

if (t_1 + t_2 > tpwm)
    t1 = (tpwm * t_1) / (t_1 + t_2);
    t2 = (tpwm * t_2) / (t_1 + t_2);
else
    t1 = t_1;
    t2 = t_2;
end

== matlab function OEW_PMSM_180_SVPWM_FOC/180_SVPWM/VSI_1/MATLAB Function ==
  data: N input; tc1 output; t1 input; t2 input; tpwm input; tc2 output; tc3 output
function [tc1,tc2,tc3] = fcn(N,t1,t2,tpwm)

ta = 0.25 * (tpwm - t1 - t2);
tb = ta + 0.5 * t1;
tc = tb + 0.5 * t2;

if N == 1
    tc1 = tb;
    tc2 = ta;
    tc3 = tc;
elseif N == 2
    tc1 = ta;
    tc2 = tc;
    tc3 = tb;
elseif N == 3
    tc1 = ta;
    tc2 = tb;
    tc3 = tc;
elseif N == 4
    tc1 = tc;
    tc2 = tb;
    tc3 = ta;
elseif N == 5
    tc1 = tc;
    tc2 = ta;
    tc3 = tb;
elseif N == 6
    tc1 = tb;
    tc2 = tc;
    tc3 = ta;
else
    tc1 = tb;
    tc2 = ta;
    tc3 = tc;
end

== matlab function OEW_PMSM_180_SVPWM_FOC/180_SVPWM/VSI_2/MATLAB Function ==
  data: N input; tc1 output; t1 input; t2 input; tpwm input; tc2 output; tc3 output
function [tc1,tc2,tc3] = fcn(N,t1,t2,tpwm)

ta = 0.25 * (tpwm - t1 - t2);
tb = ta + 0.5 * t1;
tc = tb + 0.5 * t2;

if N == 1
    tc1 = tb;
    tc2 = tc;
    tc3 = ta;
elseif N == 2
    tc1 = tc;
    tc2 = ta;
    tc3 = tb;
elseif N == 3
    tc1 = tc;
    tc2 = tb;
    tc3 = ta;
elseif N == 4
    tc1 = ta;
    tc2 = tb;
    tc3 = tc;
elseif N == 5
    tc1 = ta;
    tc2 = tc;
    tc3 = tb;
elseif N == 6
    tc1 = tb;
    tc2 = ta;
    tc3 = tc;
else
    tc1 = tb;
    tc2 = tc;
    tc3 = ta;
end
